simulink model "altitude_contr_nonlin_plant"  (R2024a)
settings: Solver=FixedStepAuto  StartTime=0.0  StopTime=SIMTIME  FixedStep=sample_time  RelTol=1e-3
undefined symbols (not defined in the file): g, J, Jr, Kd, m
settings Model: Creator=Lorenzo-Desk  LastModifiedBy=Lorenzo-Desk

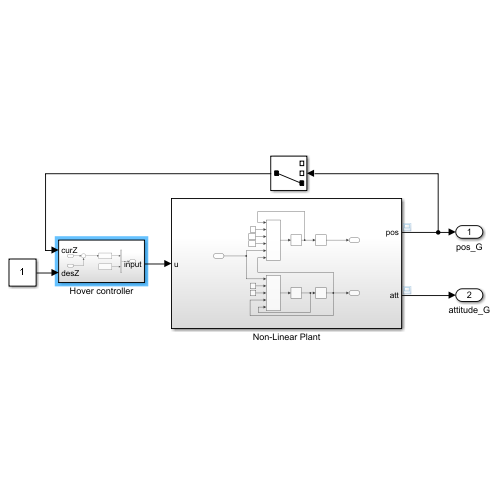
[thumbnail: Simulink's stored preview of the top-level diagram]
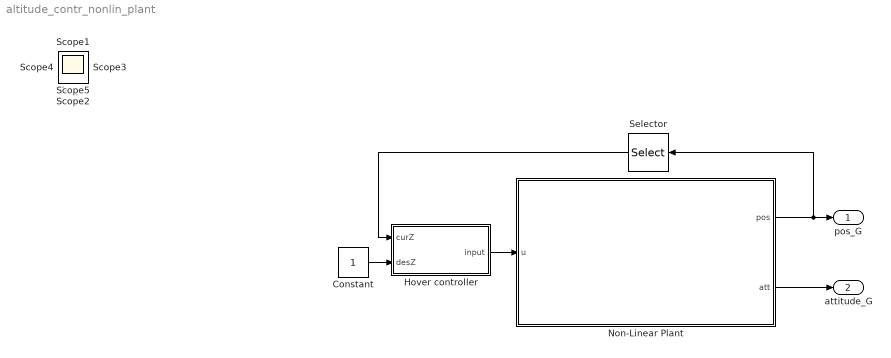
== system altitude_contr_nonlin_plant ==
  Constant : Constant
  Hover controller : Subsystem
  Non-Linear Plant : Subsystem
  Selector : Selector  InputPortWidth=3  IndexOptions=Index vector (dialog)  Indices=[3]  OutputSizes=1
  pos_G : Outport
  attitude_G : Outport  Port=2
  Scope{,1..5} (6 alike) : Scope
  wires:
  Hover controller/1(input) -> Non-Linear Plant/1(u)
  Non-Linear Plant/1(pos) -> Selector/1, pos_G/1
  Non-Linear Plant/2(att) -> attitude_G/1
  Selector/1 -> Hover controller/1(curZ)
  Constant/1 -> Hover controller/2(desZ)

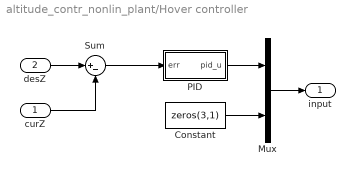
== system altitude_contr_nonlin_plant/Hover controller ==
  curZ : Inport
  desZ : Inport  Port=2
  Constant : Constant  Value=zeros(3,1)
  Mux : Mux  Inputs=2
  PID : Subsystem
  Sum : Sum  Inputs=|+-
  input : Outport
  wires:
  Sum/1 -> PID/1(err)
  Constant/1 -> Mux/2
  Mux/1 -> input/1
  desZ/1 -> Sum/1
  curZ/1 -> Sum/2
  PID/1(pid_u) -> Mux/1

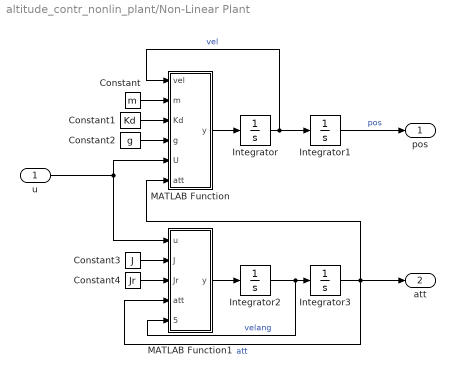
== system altitude_contr_nonlin_plant/Non-Linear Plant ==
  u : Inport  PortDimensions=4
  Constant : Constant  Value=m
  Constant1 : Constant  Value=Kd
  Constant2 : Constant  Value=g
  Constant3 : Constant  Value=J
  Constant4 : Constant  Value=Jr
  Integrator{,1..3} (4 alike) : Integrator
  MATLAB Function : MATLAB Function  TreatAsAtomicUnit=on
  MATLAB Function1 : MATLAB Function  TreatAsAtomicUnit=on
  pos : Outport  PortDimensions=3
  att : Outport  Port=2  PortDimensions=3
  wires:
  u/1 -> MATLAB Function1/1(u), MATLAB Function/5(U)
  Integrator2/1 -> MATLAB Function1/5(velang), Integrator3/1  "velang"
  Constant4/1 -> MATLAB Function1/3(Jr)
  MATLAB Function/1(y) -> Integrator/1
  Integrator/1 -> MATLAB Function/1(vel), Integrator1/1  "vel"
  Constant/1 -> MATLAB Function/2(m)
  Integrator3/1 -> MATLAB Function1/4(att), att/1, MATLAB Function/6(att)  "att"
  MATLAB Function1/1(y) -> Integrator2/1
  Integrator1/1 -> pos/1  "pos"
  Constant1/1 -> MATLAB Function/3(Kd)
  Constant2/1 -> MATLAB Function/4(g)
  Constant3/1 -> MATLAB Function1/2(J)

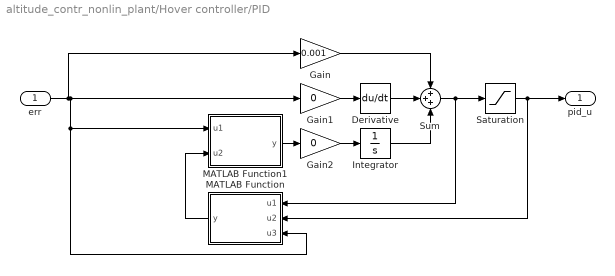
== system altitude_contr_nonlin_plant/Hover controller/PID ==
  err : Inport
  Derivative : Derivative
  Gain : Gain  Gain=0.001
  Gain1 : Gain  Gain=0
  Gain2 : Gain  Gain=0
  Integrator : Integrator
  MATLAB Function : MATLAB Function  TreatAsAtomicUnit=on
  MATLAB Function1 : MATLAB Function  TreatAsAtomicUnit=on
  Saturation : Saturate  UpperLimit=18  LowerLimit=-18
  Sum : Sum  Inputs=+++
  pid_u : Outport
  wires:
  Gain1/1 -> Derivative/1
  Gain2/1 -> Integrator/1
  Gain/1 -> Sum/1
  Derivative/1 -> Sum/2
  Integrator/1 -> Sum/3
  Sum/1 -> MATLAB Function/1(u1), Saturation/1
  Saturation/1 -> MATLAB Function/2(u2), pid_u/1
  err/1 -> Gain1/1, MATLAB Function1/1(u1), MATLAB Function/3(u3), Gain/1
  MATLAB Function1/1(y) -> Gain2/1
  MATLAB Function/1(y) -> MATLAB Function1/2(u2)

== matlab function altitude_contr_nonlin_plant/Non-Linear Plant/MATLAB Function ==
  data: vel input; m input; Kd input; g input; U input; att input; y output
function y = fcn(vel, m, Kd, g, U, att)
u = vel(1); v = vel(2); w = vel(3);
phi = att(1); theta = att(2); psi = att(3);
kdx = Kd(1); kdy = Kd(2); kdz = Kd(3);
y = zeros(3,1);
y(1) = -U(1)/m * (cos(phi)*sin(theta)*cos(psi) + sin(phi)*sin(psi)) - kdx*u;
y(2) = U(1)/m * (-cos(phi)*cos(theta)*sin(psi) + sin(phi) * cos(psi)) - kdy*v;
y(3) = -U(1)/m*cos(phi)*cos(theta) - kdz * w + g;

== matlab function altitude_contr_nonlin_plant/Hover controller/PID/MATLAB Function ==
  data: u1 input; y output; u2 input; u3 input
function y = fcn(u1, u2, u3)
if u1 ~= u2
    check1 = 0;
else
    check1 = 1;
end
if sign(u1) == sign(u3)
    check2 = 1;
else
    check2 = 0;
end
if check1 && check2
    y = 1;
else
    y = 0;
end

== matlab function altitude_contr_nonlin_plant/Non-Linear Plant/MATLAB Function1 ==
  data: u input; y output; J input; Jr input; att input; velang input
function y = fcn(u, J, Jr, att, velang)
Jx = J(1); Jy = J(2); Jz = J(3);
phi = att(1); theta = att(2); psi = att(3);
phi_dot = velang(1); theta_dot = velang(2); psi_dot = velang(3);
Rr = [1 0 -sin(theta);
      0 cos(phi) sin(phi)*cos(theta);
      0 -sin(phi) cos(phi)*cos(theta)];
b_velang = inv(Rr)*velang;
B_phi_dot = velang(1); B_theta_dot = velang(2); B_psi_dot = velang(3);

y = zeros(3,1);
y(1) = (Jy-Jz/Jx)*B_theta_dot*B_psi_dot-Jr/Jx*B_theta_dot*u(1)+u(2)/Jx;
y(2) = (Jz-Jx/Jy)*B_phi_dot*B_psi_dot+Jr/Jy*B_phi_dot*u(1)+u(3)/Jy;
y(3) = (Jx-Jy/Jz)*B_phi_dot*B_theta_dot+u(4)/Jz;

%y(1) = (Jy-Jz/Jx)*theta_dot*psi_dot-Jr/Jx*theta_dot*u(1)+u(2)/Jx;
%y(2) = (Jz-Jx/Jy)*phi_dot*psi_dot+Jr/Jy*phi_dot*u(1)+u(3)/Jy;
%y(3) = (Jx-Jy/Jz)*phi_dot*theta_dot+u(4)/Jz;

== matlab function altitude_contr_nonlin_plant/Hover controller/PID/MATLAB Function1 ==
  data: u1 input; y output; u2 input
function y = fcn(u1,u2)
if u2 == 1
    y = 0;
else
    y = u1;
end
